simulink model "part10final"  (R2017b)
settings: Solver=VariableStepAuto  StartTime=0.0  StopTime=100  RelTol=1e-3
settings Model: Creator=admin  LastModifiedBy=admin

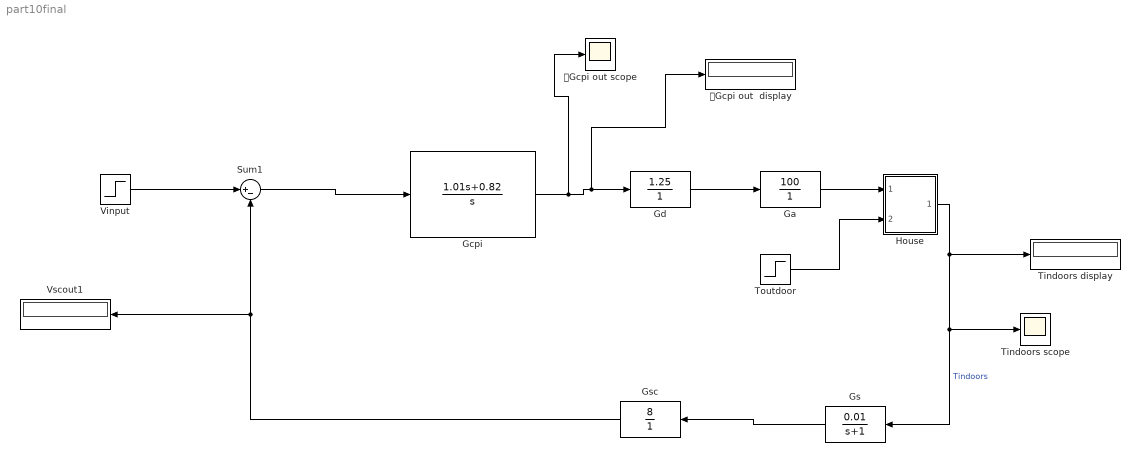
== system part10final ==
  Ga : TransferFcn  Numerator=[100]  Denominator=[1 ]
  "Gcpi " : TransferFcn  Numerator=[1.01 0.82]  Denominator=[1 0]
  "Gd " : TransferFcn  Numerator=[1.25]  Denominator=[1 ]
  "Gs " : TransferFcn  Numerator=[0.01]  Denominator=[1 1]
  Gsc : TransferFcn  Numerator=[8]  Denominator=[1 ]
  House : Subsystem
      mask Display: image(fullfile(matlabroot,'toolbox','simulink','simdemos','simgeneral','images','HouseHeatHousePix.svg'))
  Sum1 : Sum  Inputs=|+-
  "Tindoors display " : Display
  Tindoors scope : Scope
  "Toutdoor " : Step  Time=0  After=15  SampleTime=0
  Vinput : Step  Time=0  After=2.06  SampleTime=0
  "Vscout1 " : Display
  "ٖGcpi out  display " : Display
  "ٖGcpi out scope " : Scope
  wires:
  Ga/1 -> House/1(Heater QDot In)
  Vinput/1 -> Sum1/1
  "Gcpi "/1 -> "ٖGcpi out scope "/1, "ٖGcpi out  display "/1, "Gd "/1
  Gsc/1 -> "Vscout1 "/1, Sum1/2
  "Gd "/1 -> Ga/1
  House/1(Room Temp Troom) -> "Tindoors display "/1, Tindoors scope/1, "Gs "/1  "Tindoors"
  Sum1/1 -> "Gcpi "/1
  "Gs "/1 -> Gsc/1
  "Toutdoor "/1 -> House/2(Outdoor Temp Tout)

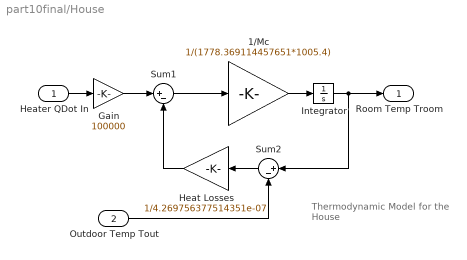
== system part10final/House ==
  note: Thermodynamic Model
      | for the House
  Heater QDot In : Inport
  Outdoor Temp Tout : Inport  Port=2
  1/Mc : Gain  Gain=1/(1778.369114457651*1005.4)  SaturateOnIntegerOverflow=on  OutDataTypeStr=Inherit: Same as input  ParamDataTypeStr=Inherit: Same as input
  Gain : Gain  Gain=100000
  Heat Losses : Gain  Gain=1/4.269756377514351e-07  SaturateOnIntegerOverflow=on  OutDataTypeStr=Inherit: Same as input  ParamDataTypeStr=Inherit: Same as input
  Integrator : Integrator  InitialCondition=20
  Sum1 : Sum  Inputs=|+-  SaturateOnIntegerOverflow=on  InputSameDT=on  OutDataTypeStr=Inherit: Same as first input
  Sum2 : Sum  Inputs=|+-  SaturateOnIntegerOverflow=on  InputSameDT=on  OutDataTypeStr=Inherit: Same as first input
  Room Temp Troom : Outport  InitialOutput=0
  wires:
  Outdoor Temp Tout/1 -> Sum2/2
  Heater QDot In/1 -> Gain/1
  Sum1/1 -> 1/Mc/1
  Sum2/1 -> Heat Losses/1
  Heat Losses/1 -> Sum1/2
  1/Mc/1 -> Integrator/1
  Integrator/1 -> Sum2/1, Room Temp Troom/1
  Gain/1 -> Sum1/1
